simulink model "lab1OrozcoBenavidesPunto3"  (R2017b)
settings: Solver=VariableStepAuto  StartTime=0.0  StopTime=0.005  RelTol=1e-3
libraries: dsparch4 x1
settings Model: Creator=user  LastModifiedBy=user

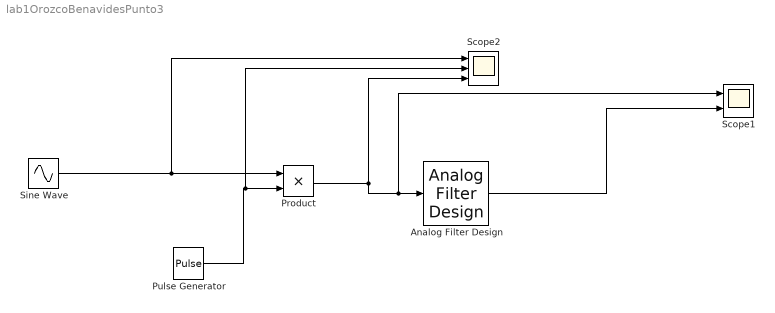
== system lab1OrozcoBenavidesPunto3 ==
  Analog Filter Design : dsparch4/Analog Filter Design  method=Butterworth  filttype=Lowpass  N=8  Wlo=2*pi*2e3  Whi=80  Rp=2  Rs=40
  Product : Product
  Pulse Generator : DiscretePulseGenerator  PulseType=Time based  Period=1/2e3  PulseWidth=50
  Scope1 : Scope  NumInputPorts=2
  Scope2 : Scope  NumInputPorts=3
  Sine Wave : Sin  Amplitude=5  Frequency=1000*2*pi  SampleTime=1/1000e3
  wires:
  Pulse Generator/1 -> Scope2/2, Product/2
  Sine Wave/1 -> Scope2/1, Product/1
  Product/1 -> Scope2/3, Scope1/1, Analog Filter Design/1
  Analog Filter Design/1 -> Scope1/2
